simulink model "LowLevelControl"  (R2017b)
settings: Solver=VariableStepAuto  StartTime=0.0  StopTime=10.0  RelTol=1e-3
values from neighbouring files (symbols this model uses):
  Bm = 0.02    [DCmotorParam.m]
  Jm = 6.8*10^(-4)    (= 0.00068)    [DCmotorParam.m]
  Kb = 0.8598    [DCmotorParam.m]
  Ki = 0.7    [DCmotorParam.m]
  La = 5.8*10^(-3)    (= 0.0058)    [DCmotorParam.m]
  Ra = 0.8    [DCmotorParam.m]
libraries: simulink x1
settings Model: Creator=Sarah Bassem  LastModifiedBy=Sarah Bassem

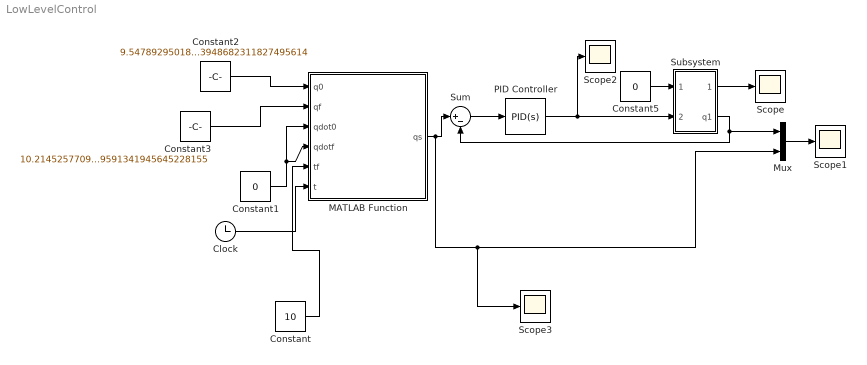
== system LowLevelControl ==
  Clock : Clock
  Constant : Constant  Value=10
  Constant1 : Constant  Value=0
  Constant2 : Constant  Value=9.5478929501873948682311827495614
  Constant3 : Constant  Value=10.214525770989591341945645228155
  Constant5 : Constant  Value=0
  MATLAB Function : MATLAB Function  TreatAsAtomicUnit=on
  Mux : Mux  Inputs=2
  PID Controller : simulink/Continuous/PID Controller  Controller=PID  TimeDomain=Continuous-time  SampleTime=-1  IntegratorMethod=Forward Euler  FilterMethod=Forward Euler  Form=Parallel  UseFilter=on  ControllerParametersSource=internal  P=1.3  I=1.2  D=3.8  N=269.212074594425  InitialConditionSource=internal  InitialConditionForIntegrator=0  InitialConditionForFilter=0  ExternalReset=none  LimitOutput=off  UpperSaturationLimit=inf  LowerSaturationLimit=-inf  LinearizeAsGain=on  AntiWindupMode=none  Kb=1  TrackingMode=off  Kt=1  PParamMin=[]  PParamMax=[]  IParamMin=[]  IParamMax=[]  DParamMin=[]  DParamMax=[]  NParamMin=[]  NParamMax=[]  KbParamMin=[]  KbParamMax=[]  KtParamMin=[]  KtParamMax=[]  POutMin=[]  POutMax=[]  IOutMin=[]  IOutMax=[]  DOutMin=[]  DOutMax=[]  NOutMin=[]  NOutMax=[]  KbOutMin=[]  KbOutMax=[]  KtOutMin=[]  KtOutMax=[]  IntegratorOutMin=[]  IntegratorOutMax=[]  FilterOutMin=[]  FilterOutMax=[]  SumOutMin=[]  SumOutMax=[]  SumI1OutMin=[]  SumI1OutMax=[]  SumI2OutMin=[]  SumI2OutMax=[]  SumI3OutMin=[]  SumI3OutMax=[]  SumDOutMin=[]  SumDOutMax=[]  SaturationOutMin=[]  SaturationOutMax=[]  IntegratorContinuousStateAttributes=''  IntegratorStateMustResolveToSignalObject=off  IntegratorRTWStateStorageClass=Auto  FilterContinuousStateAttributes=''  FilterStateMustResolveToSignalObject=off  FilterRTWStateStorageClass=Auto  DifferentiatorICPrevScaledInput=0  DifferentiatorOutMin=[]  DifferentiatorOutMax=[]  InitialConditionSetting=State (most efficient)  FilterDiffOutCoefMin=[]  FilterDiffOutCoefMax=[]  SumDenOutMin=[]  SumDenOutMax=[]  SumNumOutMin=[]  SumNumOutMax=[]  ReciprocalOutMin=[]  ReciprocalOutMax=[]  DivideOutMin=[]  DivideOutMax=[]  TunerSelectOption=Transfer Function Based (PID Tuner App)
  Scope{,1..3} (4 alike) : Scope
  Subsystem : Subsystem
  Sum : Sum  Inputs=|+-
  wires:
  Constant5/1 -> Subsystem/1(In1)
  Subsystem/1(q1dot) -> Scope/1
  PID Controller/1 -> Scope2/1, Subsystem/2(In2)
  Sum/1 -> PID Controller/1
  MATLAB Function/1(qs) -> Sum/1, Scope3/1, Mux/2
  Mux/1 -> Scope1/1
  Subsystem/2(q1) -> Mux/1, Sum/2
  Constant/1 -> MATLAB Function/5(tf)
  Constant1/1 -> MATLAB Function/3(qdot0), MATLAB Function/4(qdotf)
  Constant3/1 -> MATLAB Function/2(qf)
  Constant2/1 -> MATLAB Function/1(q0)
  Clock/1 -> MATLAB Function/6(t)

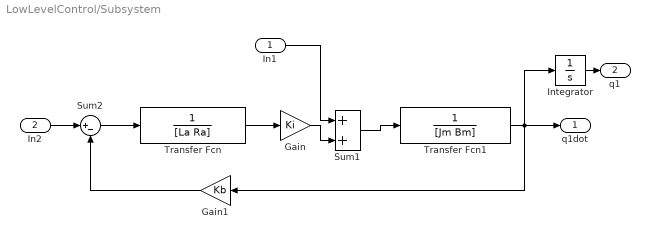
== system LowLevelControl/Subsystem ==
  In1 : Inport
  In2 : Inport  Port=2
  Gain : Gain  Gain=Ki
  Gain1 : Gain  Gain=Kb
  Integrator : Integrator
  Sum1 : Sum
  Sum2 : Sum  Inputs=|+-
  Transfer Fcn : TransferFcn  Denominator=[La Ra]
  Transfer Fcn1 : TransferFcn  Denominator=[Jm Bm]
  q1dot : Outport
  q1 : Outport  Port=2
  wires:
  In2/1 -> Sum2/1
  Transfer Fcn/1 -> Gain/1
  Gain1/1 -> Sum2/2
  Sum2/1 -> Transfer Fcn/1
  Gain/1 -> Sum1/2
  Sum1/1 -> Transfer Fcn1/1
  In1/1 -> Sum1/1
  Transfer Fcn1/1 -> Gain1/1, Integrator/1, q1dot/1
  Integrator/1 -> q1/1

== matlab function LowLevelControl/MATLAB Function ==
  data: q0 input; qs output; qf input; qdot0 input; qdotf input; tf input; t input
function qs = Reference(q0, qf, qdot0, qdotf, tf,t)
coder.extrinsic('joint_traj_first_joint');
%q1=zeros(100,1);
qs=0;
qs=joint_traj_first_joint(q0, qf, qdot0, qdotf, tf,t);
% i=1;
% for t=0.1:0.1:tf
%    q1=qs(i,1);
%    i=i+1;
% end
%q1=qs(:,1);
% i=1;
% for t=0:0.1:10
%     if t==0
%         q1=10;
%     else
%     q1=q1s(i);
%     i=i+1;
%     end
%  end
end
